simulink model "ap_12BAdapted_with_contracts_AutoPilot"  (R2017b)
settings: Solver=FixedStepDiscrete  StartTime=0.0  StopTime=500  FixedStep=Ts  RelTol=1e-3  EnableMultiTasking=on
undefined symbols (not defined in the file): beaver_b, beaver_c, beaver_mass, beaver_S, Cl0, Cl_alpha2_dpt, Cl_beta, Cl_da, Cl_da_alpha, Cl_dr, Cl_p, Cl_r, Cm0, Cm_alpha, Cm_alpha2, Cm_beta2, Cm_de, Cm_df, Cm_dpt, Cm_q, Cm_r, Cn0, Cn_beta, Cn_beta3, Cn_da, Cn_dpt3, Cn_dr, Cn_p, Cn_q, Cn_r, contractAfterSimulation, contractBeforeSimulation, ContractBlock, ContractEnsureBlock, ContractGuaranteeBlock, ContractModeBlock, ContractRequireBlock, ContractValidatorBlock, Cx0, Cx_alpha, Cx_alpha2, Cx_alpha3, Cx_df, Cx_df_alpha, Cx_dpt, Cx_dpt2_alpha, Cx_dr, Cx_q, Cy0, Cy_beta, Cy_da, Cy_dr, Cy_dr_alpha, Cy_p, Cy_r, Cz0, Cz_alpha, Cz_alpha3, Cz_de, Cz_de_beta ... (+32)
libraries: simulink x10, cocosimLibs x3
(part 3 of 4)

== system ap_12BAdapted_with_contracts_AutoPilot/GlobalScope/DeHavilland Beaver Airframe/Aircraft Dynamics/6DoF (Quaternion)/Calculate DCM & Euler Angles/Quaternions to Direction Cosine Matrix ==
  Quat : Inport  Unit=1  PortDimensions=4
  A11 : Subsystem
  A12 : Subsystem
  A13 : Subsystem
  A21 : Subsystem
  A22 : Subsystem
  A23 : Subsystem
  A31 : Subsystem
  A32 : Subsystem
  A33 : Subsystem
  Create 3x3 Matrix : Subsystem  mask(Create 3x3 Matrix){}
      mask help: shared_aeroblks:sharedaeroblkutil:blockCreate3x3MatrixDesc
      mask init:
      | if license('test','aerospace_blockset')
      |     aerosharedicon('shared');
      | elseif license('test','powertrain_blockset')
      |     sharedautoicon('shared');
      | end
      mask Help: eval('if license(''test'',''aerospace_blockset'')aerosharedhelp(''create_threebythree_matrix'');elseif license(''test'',''powertrain_blockset'')sharedautohelp(''create_threebythree_matrix'');end')
      mask Display:
      | port_label('input',1,'A_{11}','texmode','on');
      | port_label('input',2,'A_{12}','texmode','on');
      | port_label('input',3,'A_{13}','texmode','on');
      | port_label('input',4,'A_{21}','texmode','on');
      | port_label('input',5,'A_{22}','texmode','on');
      | port_label('input',6,'A_{23}','texmode','on');
      | port_label('input',7,'A_{31}','texmode','on');
      | port_label('input',8,'A_{32}','texmode','on');
      | port_label('input',9,'A_{33}','texmode','on');
      | port_label('output',1,'A','texmode','on');
  Quaternion Normalize : Subsystem  mask(Quaternion Normalize){}
      mask help: shared_aeroblks:sharedaeroblkutil:blockQuaternionNormalizeDesc
      mask init:
      | if license('test','aerospace_blockset')
      |     aerosharedicon('shared');
      | elseif license('test','powertrain_blockset')
      |     sharedautoicon('shared');
      | end
      mask Help: eval('if license(''test'',''aerospace_blockset'')aerosharedhelp;elseif license(''test'',''powertrain_blockset'')sharedautohelp;end')
  DCM : Outport  Unit=1  PortDimensions=[3,3]  VectorParamsAs1DForOutWhenUnconnected=off
  wires:
  A21/1(A21) -> Create 3x3 Matrix/4(M21)
  A12/1(A12) -> Create 3x3 Matrix/2(M12)
  Create 3x3 Matrix/1(Matrix) -> DCM/1
  A22/1(A22) -> Create 3x3 Matrix/5(M22)
  A32/1(A32) -> Create 3x3 Matrix/8(M32)
  A33/1(A33) -> Create 3x3 Matrix/9(M33)
  A31/1(A31) -> Create 3x3 Matrix/7(M31)
  A11/1(A11) -> Create 3x3 Matrix/1(M11)
  A13/1(A13) -> Create 3x3 Matrix/3(M13)
  A23/1(A23) -> Create 3x3 Matrix/6(M23)
  Quaternion Normalize/1(normal(q)) -> A11/1(normal(q)), A12/1(normal(q)), A13/1(normal(q)), A21/1(normal(q)), A22/1(normal(q)), A23/1(normal(q)), A31/1(normal(q)), A32/1(normal(q)), A33/1(normal(q))
  Quat/1 -> Quaternion Normalize/1(q)

== system ap_12BAdapted_with_contracts_AutoPilot/GlobalScope/DeHavilland Beaver Airframe/Aircraft Dynamics/6DoF (Quaternion)/Calculate DCM & Euler Angles/Quaternions to Rotation Angles (ZYX) ==
  q : Inport
  Quaternion Normalize : Subsystem
  Trigonometric Function1 : Trigonometry  Operator=atan2
  Trigonometric Function3 : Trigonometry  Operator=atan2
  Vector Concatenate : Concatenate  NumInputs=3
  fcn1 : Fcn  Expr=2*(u[2]*u[3] + u[1]*u[4])
  fcn2 : Fcn  Expr=u[1]*u[1] + u[2]*u[2] - u[3]*u[3] - u[4]*u[4]
  fcn3 : Fcn  Expr=-2*(u[2]*u[4] - u[1]*u[3])
  fcn4 : Fcn  Expr=2*(u[3]*u[4] + u[1]*u[2])
  fcn5 : Fcn  Expr=u[1]*u[1] - u[2]*u[2] - u[3]*u[3] + u[4]*u[4]
  trigFcn : Trigonometry  Operator=asin
  R1,R2,R3 : Outport  VectorParamsAs1DForOutWhenUnconnected=off
  wires:
  fcn5/1 -> Trigonometric Function3/2
  fcn4/1 -> Trigonometric Function3/1
  fcn2/1 -> Trigonometric Function1/2
  fcn3/1 -> trigFcn/1
  q/1 -> Quaternion Normalize/1(q)
  Vector Concatenate/1 -> R1,R2,R3/1
  Trigonometric Function3/1 -> Vector Concatenate/3  "r3"
  Trigonometric Function1/1 -> Vector Concatenate/1  "r1"
  Quaternion Normalize/1(normal(q)) -> fcn1/1, fcn2/1, fcn5/1, fcn4/1, fcn3/1
  trigFcn/1 -> Vector Concatenate/2  "r2"
  fcn1/1 -> Trigonometric Function1/1

== system ap_12BAdapted_with_contracts_AutoPilot/GlobalScope/DeHavilland Beaver Airframe/Aircraft Dynamics/6DoF (Quaternion)/Calculate DCM & Euler Angles/ResetIntegratorInternal1 ==
  note: ic
  note: Level Reset Integration With Saturation
      | y(n) = y(n-1) + K*Ts*u(n-1)
  U : Inport
  R : Inport  Port=2
  IC : Inport  Port=3
  Constant : Constant  Value=1.0
  Constant1 : Constant  Value=Ts
  Product : Product  RndMeth=Zero
  Product1 : Product  RndMeth=Zero
  Saturation : Saturate  UpperLimit=20  LowerLimit=-20
  Sum3 : Sum
  Switch : Switch  Criteria=u2 ~= 0
  Switch1 : Switch  Criteria=u2 ~= 0
  X : UnitDelay  SampleTime=Ts  HasFrameUpgradeWarning=on
  Y : Outport  VectorParamsAs1DForOutWhenUnconnected=off
  wires:
  Product1/1 -> Sum3/1
  U/1 -> Product1/2
  Sum3/1 -> Switch1/3
  Product/1 -> Product1/1
  Switch/1 -> Saturation/1
  IC/1 -> Switch1/1, Switch/1
  Constant1/1 -> Product/2  "deltaT"
  Switch1/1 -> X/1
  Constant/1 -> Product/1  "gain"
  Saturation/1 -> Y/1, Sum3/2
  R/1 -> Switch1/2, Switch/2
  X/1 -> Switch/3

== system ap_12BAdapted_with_contracts_AutoPilot/GlobalScope/DeHavilland Beaver Airframe/Aircraft Dynamics/6DoF (Quaternion)/Calculate DCM & Euler Angles/Rotation Angles to Quats (ZYX) ==
  "R1, R2, R3" : Inport
  1/2 : Gain  Gain=0.5  SaturateOnIntegerOverflow=on  OutDataTypeStr=Inherit: Same as input  ParamDataTypeStr=Inherit: Same as input
  Mux1 : Mux  Inputs=2
  Mux2 : Mux
  q0 : Fcn  Expr=u(4)*u(5)*u(6) + u(1)*u(2)*u(3)
  q1 : Fcn  Expr=u(4)*u(5)*u(3) - u(1)*u(2)*u(6)
  q2 : Fcn  Expr=u(4)*u(2)*u(6) + u(1)*u(5)*u(3)
  q3 : Fcn  Expr=u(1)*u(5)*u(6) - u(4)*u(2)*u(3)
  sincos : Trigonometry  Operator=sincos
  Quat : Outport  VectorParamsAs1DForOutWhenUnconnected=off
  wires:
  sincos/1 -> Mux1/1
  1/2/1 -> sincos/1
  "R1, R2, R3"/1 -> 1/2/1
  sincos/2 -> Mux1/2
  Mux1/1 -> q0/1, q1/1, q2/1, q3/1
  q1/1 -> Mux2/2
  q2/1 -> Mux2/3
  q3/1 -> Mux2/4
  Mux2/1 -> Quat/1
  q0/1 -> Mux2/1

== system ap_12BAdapted_with_contracts_AutoPilot/GlobalScope/DeHavilland Beaver Airframe/Aircraft Dynamics/6DoF (Quaternion)/Calculate DCM & Euler Angles/ic3 ==
  ic : Inport
  Constant : Constant  Value=0
  Unit Delay : UnitDelay  InitialCondition=1  SampleTime=-1  HasFrameUpgradeWarning=on
  R : Outport  VectorParamsAs1DForOutWhenUnconnected=off
  IC : Outport  Port=2  VectorParamsAs1DForOutWhenUnconnected=off
  wires:
  Constant/1 -> Unit Delay/1
  Unit Delay/1 -> R/1
  ic/1 -> IC/1

== system ap_12BAdapted_with_contracts_AutoPilot/GlobalScope/DeHavilland Beaver Airframe/Aircraft Dynamics/6DoF (Quaternion)/Calculate DCM & Euler Angles/qd ==
  p q r : Inport
  q0 q1 q2 q3 : Inport  Port=2
  Constant : Constant
  Dot Product : DotProduct  OutDataTypeStr=Inherit: Inherit via internal rule
  High Gain Quaternion Normalization : Gain  Gain=1.0  SaturateOnIntegerOverflow=on  OutDataTypeStr=Inherit: Same as input  ParamDataTypeStr=Inherit: Same as input
  Mux1 : Mux  Inputs=[3 4 1]
  Mux2 : Mux
  Sum : Sum  Inputs=|+-  SaturateOnIntegerOverflow=on  InputSameDT=on  OutDataTypeStr=Inherit: Same as first input
  q0dot : Fcn  Expr=-0.5 * ( u[5]*u[1]+u[6]*u[2]+u[7]*u[3] ) + u[8]*u[4]
  q1dot : Fcn  Expr=0.5 * ( u[4]*u[1]+u[6]*u[3]-u[7]*u[2] ) + u[8]*u[5]
  q2dot : Fcn  Expr=0.5 * ( u[4]*u[2]+u[7]*u[1]-u[5]*u[3] ) + u[8]*u[6]
  q3dot : Fcn  Expr=0.5 * ( u[4]*u[3]+u[5]*u[2]-u[6]*u[1] ) + u[8]*u[7]
  qdot : Outport  VectorParamsAs1DForOutWhenUnconnected=off
  wires:
  p q r/1 -> Mux1/1
  q3dot/1 -> Mux2/4
  q2dot/1 -> Mux2/3
  q1dot/1 -> Mux2/2
  Constant/1 -> Sum/1
  Mux1/1 -> q2dot/1, q3dot/1, q0dot/1, q1dot/1
  q0dot/1 -> Mux2/1
  Mux2/1 -> qdot/1
  Sum/1 -> High Gain Quaternion Normalization/1
  Dot Product/1 -> Sum/2
  High Gain Quaternion Normalization/1 -> Mux1/3
  q0 q1 q2 q3/1 -> Dot Product/1, Dot Product/2, Mux1/2

== system ap_12BAdapted_with_contracts_AutoPilot/GlobalScope/DeHavilland Beaver Airframe/Aircraft Dynamics/6DoF (Quaternion)/Calculate omega_dot/3x3 CrossProduct ==
  A : Inport
  B : Inport  Port=2
  "A " : InportShadow
  "B " : InportShadow  Port=2
  Subsystem : Subsystem
  Subsystem1 : Subsystem
  Sum : Sum  Inputs=+|-  SaturateOnIntegerOverflow=on  InputSameDT=on  OutDataTypeStr=Inherit: Same as first input
  C : Outport  VectorParamsAs1DForOutWhenUnconnected=off
  wires:
  "A "/1 -> Subsystem1/1(A)
  Subsystem/1(Out1) -> Sum/1
  B/1 -> Subsystem/2(B)
  Sum/1 -> C/1
  "B "/1 -> Subsystem1/2(B)
  Subsystem1/1(Out1) -> Sum/2
  A/1 -> Subsystem/1(A)

== system ap_12BAdapted_with_contracts_AutoPilot/GlobalScope/DeHavilland Beaver Airframe/Aircraft Dynamics/6DoF (Quaternion)/Calculate omega_dot/I x w ==
  p q r : Inport
  Inertia : Inport  Port=2
  Product : Product  Multiplication=Matrix(*)  SaturateOnIntegerOverflow=on  InputSameDT=on  OutDataTypeStr=Inherit: Same as first input
  Reshape1 : Reshape  OutputDimensionality=Column vector (2-D)
  Reshape2 : Reshape
  I * w : Outport  VectorParamsAs1DForOutWhenUnconnected=off
  wires:
  Reshape2/1 -> I * w/1
  Reshape1/1 -> Product/2
  p q r/1 -> Reshape1/1
  Inertia/1 -> Product/1
  Product/1 -> Reshape2/1

== system ap_12BAdapted_with_contracts_AutoPilot/GlobalScope/DeHavilland Beaver Airframe/Aircraft Dynamics/6DoF (Quaternion)/Calculate omega_dot/I x w1 ==
  I_dot : Inport
  p q r : Inport  Port=2
  Product : Product  Multiplication=Matrix(*)  SaturateOnIntegerOverflow=on  InputSameDT=on  OutDataTypeStr=Inherit: Same as first input
  Reshape1 : Reshape  OutputDimensionality=Column vector (2-D)
  Reshape2 : Reshape
  Id * w : Outport  VectorParamsAs1DForOutWhenUnconnected=off
  wires:
  Reshape2/1 -> Id * w/1
  Reshape1/1 -> Product/2
  Product/1 -> Reshape2/1
  I_dot/1 -> Product/1
  p q r/1 -> Reshape1/1

== system ap_12BAdapted_with_contracts_AutoPilot/GlobalScope/DeHavilland Beaver Airframe/Aircraft Dynamics/Total Forces and Moments/Actuators/sof ==
  Ac_dem : Inport
  2*zeta * wn : Gain  Gain=2.0 * z_fin* wn_fin  SaturateOnIntegerOverflow=on  OutDataTypeStr=Inherit: Same as input  ParamDataTypeStr=Inherit: Same as input
  Demand limits : Saturate  UpperLimit=fin_max  LowerLimit=fin_min
  ResetIntegratorInternal : Subsystem
  ResetIntegratorInternal1 : Subsystem
  Sum2 : Sum  Inputs=|+-  SaturateOnIntegerOverflow=on  InputSameDT=on  OutDataTypeStr=Inherit: Same as first input
  Sum3 : Sum  Inputs=|+-  SaturateOnIntegerOverflow=on  InputSameDT=on  OutDataTypeStr=Inherit: Same as first input
  ic1 : Subsystem
  ic3 : Subsystem
  rate limit*2*zeta/wn : Saturate  UpperLimit=fin_maxrate*2*z_fin/wn_fin  LowerLimit=-fin_maxrate*2*z_fin/wn_fin
  wn^2 : Gain  Gain=wn_fin* wn_fin  SaturateOnIntegerOverflow=on  OutDataTypeStr=Inherit: Same as input  ParamDataTypeStr=Inherit: Same as input
  Ac_ac : Outport  VectorParamsAs1DForOutWhenUnconnected=off
  wires:
  ResetIntegratorInternal1/1(Y) -> Ac_ac/1, Sum3/2
  wn^2/1 -> Sum2/1
  ResetIntegratorInternal/1(Y) -> ResetIntegratorInternal1/1(U), 2*zeta * wn/1
  Sum2/1 -> ResetIntegratorInternal/1(U)
  Demand limits/1 -> Sum3/1
  rate limit*2*zeta/wn/1 -> wn^2/1
  Ac_dem/1 -> Demand limits/1
  Sum3/1 -> rate limit*2*zeta/wn/1
  2*zeta * wn/1 -> Sum2/2
  ic3/2(IC) -> ResetIntegratorInternal/3(ic)
  ic3/1(R) -> ResetIntegratorInternal/2(R)
  ic1/1(R) -> ResetIntegratorInternal1/2(R)
  ic1/2(IC) -> ResetIntegratorInternal1/3(ic)

== system ap_12BAdapted_with_contracts_AutoPilot/GlobalScope/DeHavilland Beaver Airframe/Aircraft Dynamics/Total Forces and Moments/Actuators/sof1 ==
  Ac_dem : Inport
  2*zeta * wn : Gain  Gain=2.0 * z_fin* wn_fin  SaturateOnIntegerOverflow=on  OutDataTypeStr=Inherit: Same as input  ParamDataTypeStr=Inherit: Same as input
  Demand limits : Saturate  UpperLimit=fin_max  LowerLimit=fin_min
  ResetIntegratorInternal : Subsystem
  ResetIntegratorInternal1 : Subsystem
  Sum2 : Sum  Inputs=|+-  SaturateOnIntegerOverflow=on  InputSameDT=on  OutDataTypeStr=Inherit: Same as first input
  Sum3 : Sum  Inputs=|+-  SaturateOnIntegerOverflow=on  InputSameDT=on  OutDataTypeStr=Inherit: Same as first input
  ic1 : Subsystem
  ic3 : Subsystem
  rate limit*2*zeta/wn : Saturate  UpperLimit=fin_maxrate*2*z_fin/wn_fin  LowerLimit=-fin_maxrate*2*z_fin/wn_fin
  wn^2 : Gain  Gain=wn_fin* wn_fin  SaturateOnIntegerOverflow=on  OutDataTypeStr=Inherit: Same as input  ParamDataTypeStr=Inherit: Same as input
  Ac_ac : Outport  VectorParamsAs1DForOutWhenUnconnected=off
  wires:
  ic1/2(IC) -> ResetIntegratorInternal1/3(ic)
  ic1/1(R) -> ResetIntegratorInternal1/2(R)
  ic3/1(R) -> ResetIntegratorInternal/2(R)
  ic3/2(IC) -> ResetIntegratorInternal/3(ic)
  2*zeta * wn/1 -> Sum2/2
  Sum3/1 -> rate limit*2*zeta/wn/1
  Ac_dem/1 -> Demand limits/1
  rate limit*2*zeta/wn/1 -> wn^2/1
  Demand limits/1 -> Sum3/1
  Sum2/1 -> ResetIntegratorInternal/1(U)
  ResetIntegratorInternal/1(Y) -> 2*zeta * wn/1, ResetIntegratorInternal1/1(U)
  wn^2/1 -> Sum2/1
  ResetIntegratorInternal1/1(Y) -> Sum3/2, Ac_ac/1

== system ap_12BAdapted_with_contracts_AutoPilot/GlobalScope/DeHavilland Beaver Airframe/Aircraft Dynamics/Total Forces and Moments/Actuators/sof2 ==
  Ac_dem : Inport
  2*zeta * wn : Gain  Gain=2.0 * z_fin* wn_fin  SaturateOnIntegerOverflow=on  OutDataTypeStr=Inherit: Same as input  ParamDataTypeStr=Inherit: Same as input
  Demand limits : Saturate  UpperLimit=fin_max  LowerLimit=fin_min
  ResetIntegratorInternal : Subsystem
  ResetIntegratorInternal1 : Subsystem
  Sum2 : Sum  Inputs=|+-  SaturateOnIntegerOverflow=on  InputSameDT=on  OutDataTypeStr=Inherit: Same as first input
  Sum3 : Sum  Inputs=|+-  SaturateOnIntegerOverflow=on  InputSameDT=on  OutDataTypeStr=Inherit: Same as first input
  ic1 : Subsystem
  ic3 : Subsystem
  rate limit*2*zeta/wn : Saturate  UpperLimit=fin_maxrate*2*z_fin/wn_fin  LowerLimit=-fin_maxrate*2*z_fin/wn_fin
  wn^2 : Gain  Gain=wn_fin* wn_fin  SaturateOnIntegerOverflow=on  OutDataTypeStr=Inherit: Same as input  ParamDataTypeStr=Inherit: Same as input
  Ac_ac : Outport  VectorParamsAs1DForOutWhenUnconnected=off
  wires:
  ResetIntegratorInternal1/1(Y) -> Ac_ac/1, Sum3/2
  wn^2/1 -> Sum2/1
  ResetIntegratorInternal/1(Y) -> ResetIntegratorInternal1/1(U), 2*zeta * wn/1
  Sum2/1 -> ResetIntegratorInternal/1(U)
  Demand limits/1 -> Sum3/1
  rate limit*2*zeta/wn/1 -> wn^2/1
  Ac_dem/1 -> Demand limits/1
  Sum3/1 -> rate limit*2*zeta/wn/1
  2*zeta * wn/1 -> Sum2/2
  ic3/2(IC) -> ResetIntegratorInternal/3(ic)
  ic3/1(R) -> ResetIntegratorInternal/2(R)
  ic1/1(R) -> ResetIntegratorInternal1/2(R)
  ic1/2(IC) -> ResetIntegratorInternal1/3(ic)

== system ap_12BAdapted_with_contracts_AutoPilot/GlobalScope/DeHavilland Beaver Airframe/Aircraft Dynamics/Total Forces and Moments/Aerodynamics/Actuator Increments ==
  alpha : Inport
  beta : Inport  Port=2
  Actuator Deflections : Inport  Port=3
  Aileron : Subsystem
  Elevator : Subsystem
  Flap : Subsystem
  Rudder : Subsystem
  Sum1 : Sum  SaturateOnIntegerOverflow=on
  Sum2 : Sum  SaturateOnIntegerOverflow=on
  Sum3 : Sum  SaturateOnIntegerOverflow=on
  Coefficients : Outport  VectorParamsAs1DForOutWhenUnconnected=off
  wires:
  Actuator Deflections/1 -> Flap/2(Actuators), Aileron/2(Actuators), Elevator/1(Actuators), Rudder/2(Actuators)
  alpha/1 -> Flap/1(Alpha), Rudder/1(Alpha), Aileron/1(alpha)
  beta/1 -> Elevator/2(Beta)
  Aileron/1(delCoeff) -> Sum1/1
  Elevator/1(delCoeff) -> Sum1/2
  Rudder/1(delCoeff) -> Sum2/2
  Flap/1(delCoeff) -> Sum3/2
  Sum3/1 -> Coefficients/1
  Sum1/1 -> Sum2/1
  Sum2/1 -> Sum3/1

== system ap_12BAdapted_with_contracts_AutoPilot/GlobalScope/DeHavilland Beaver Airframe/Aircraft Dynamics/Total Forces and Moments/Aerodynamics/Body Rate Damping ==
  V : Inport
  p,q,r : Inport  Port=2
  Demux : Demux  Outputs=3
  Product : Product  SaturateOnIntegerOverflow=on  InputSameDT=on  OutDataTypeStr=Inherit: Same as first input
  Product1 : Product  SaturateOnIntegerOverflow=on  InputSameDT=on  OutDataTypeStr=Inherit: Same as first input
  Product2 : Product  SaturateOnIntegerOverflow=on  InputSameDT=on  OutDataTypeStr=Inherit: Same as first input
  Product3 : Product  Inputs=*/  SaturateOnIntegerOverflow=on  InputSameDT=on  OutDataTypeStr=Inherit: Same as first input
  Reference Length : Gain  Gain=beaver_c  SaturateOnIntegerOverflow=on  OutDataTypeStr=Inherit: Same as input  ParamDataTypeStr=Inherit: Same as input
  Reference Span : Gain  Gain=beaver_b/2  SaturateOnIntegerOverflow=on  OutDataTypeStr=Inherit: Same as input  ParamDataTypeStr=Inherit: Same as input
  "Reference Span " : Gain  Gain=beaver_b/2  SaturateOnIntegerOverflow=on  OutDataTypeStr=Inherit: Same as input  ParamDataTypeStr=Inherit: Same as input
  Sum1 : Sum  SaturateOnIntegerOverflow=on
  Sum2 : Sum  SaturateOnIntegerOverflow=on
  p : Subsystem
  q : Subsystem
  r : Subsystem
  Coefficients : Outport  VectorParamsAs1DForOutWhenUnconnected=off
  wires:
  p/1(delCoeff) -> Product/1
  q/1(delCoeff) -> Product1/1
  p,q,r/1 -> Demux/1
  Demux/1 -> Product/2  "p"
  Demux/2 -> Product1/2  "q"
  Demux/3 -> Product2/2  "r"
  Sum1/1 -> Product3/1
  V/1 -> Product3/2
  Product3/1 -> Coefficients/1
  Product1/1 -> Reference Length/1
  Product2/1 -> "Reference Span "/1
  Product/1 -> Reference Span/1
  r/1(delCoeff) -> Product2/1
  Reference Length/1 -> Sum2/2
  "Reference Span "/1 -> Sum1/2
  Reference Span/1 -> Sum2/1
  Sum2/1 -> Sum1/1

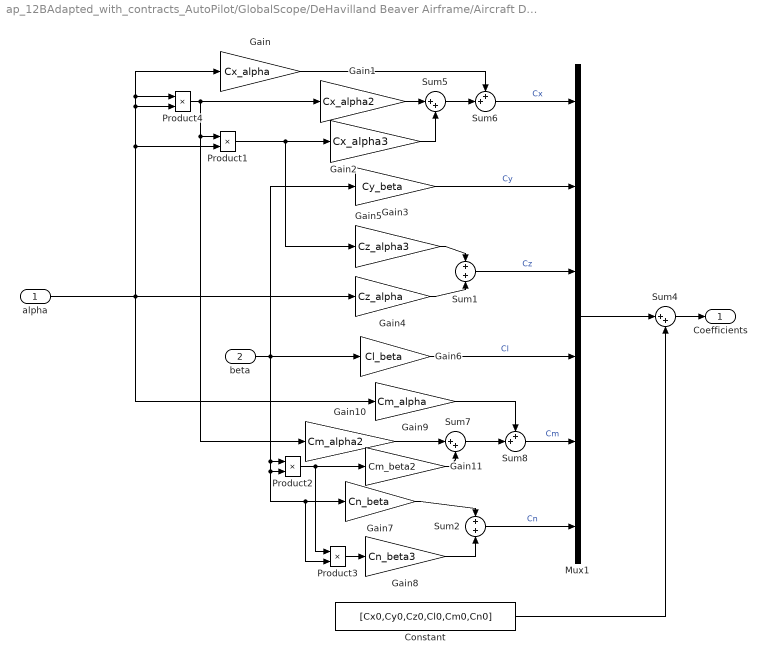
== system ap_12BAdapted_with_contracts_AutoPilot/GlobalScope/DeHavilland Beaver Airframe/Aircraft Dynamics/Total Forces and Moments/Aerodynamics/Datum Coefficients ==
  alpha : Inport
  beta : Inport  Port=2
  Constant : Constant  Value=[Cx0,Cy0,Cz0,Cl0,Cm0,Cn0]
  Gain : Gain  Gain=Cx_alpha  SaturateOnIntegerOverflow=on  OutDataTypeStr=Inherit: Same as input  ParamDataTypeStr=Inherit: Same as input
  Gain1 : Gain  Gain=Cx_alpha2  SaturateOnIntegerOverflow=on  OutDataTypeStr=Inherit: Same as input  ParamDataTypeStr=Inherit: Same as input
  Gain10 : Gain  Gain=Cm_alpha2  SaturateOnIntegerOverflow=on  OutDataTypeStr=Inherit: Same as input  ParamDataTypeStr=Inherit: Same as input
  Gain11 : Gain  Gain=Cm_beta2  SaturateOnIntegerOverflow=on  OutDataTypeStr=Inherit: Same as input  ParamDataTypeStr=Inherit: Same as input
  Gain2 : Gain  Gain=Cx_alpha3  SaturateOnIntegerOverflow=on  OutDataTypeStr=Inherit: Same as input  ParamDataTypeStr=Inherit: Same as input
  Gain3 : Gain  Gain=Cy_beta  SaturateOnIntegerOverflow=on  OutDataTypeStr=Inherit: Same as input  ParamDataTypeStr=Inherit: Same as input
  Gain4 : Gain  Gain=Cz_alpha  SaturateOnIntegerOverflow=on  OutDataTypeStr=Inherit: Same as input  ParamDataTypeStr=Inherit: Same as input
  Gain5 : Gain  Gain=Cz_alpha3  SaturateOnIntegerOverflow=on  OutDataTypeStr=Inherit: Same as input  ParamDataTypeStr=Inherit: Same as input
  Gain6 : Gain  Gain=Cl_beta  SaturateOnIntegerOverflow=on  OutDataTypeStr=Inherit: Same as input  ParamDataTypeStr=Inherit: Same as input
  Gain7 : Gain  Gain=Cn_beta  SaturateOnIntegerOverflow=on  OutDataTypeStr=Inherit: Same as input  ParamDataTypeStr=Inherit: Same as input
  Gain8 : Gain  Gain=Cn_beta3  SaturateOnIntegerOverflow=on  OutDataTypeStr=Inherit: Same as input  ParamDataTypeStr=Inherit: Same as input
  Gain9 : Gain  Gain=Cm_alpha  SaturateOnIntegerOverflow=on  OutDataTypeStr=Inherit: Same as input  ParamDataTypeStr=Inherit: Same as input
  Mux1 : Mux  Inputs=6
  Product{1..4} (4 alike) : Product  SaturateOnIntegerOverflow=on  InputSameDT=on  OutDataTypeStr=Inherit: Same as first input
  Sum1 : Sum  SaturateOnIntegerOverflow=on
  Sum2 : Sum  SaturateOnIntegerOverflow=on
  Sum4 : Sum  Inputs=|++  SaturateOnIntegerOverflow=on
  Sum5 : Sum  Inputs=|++  SaturateOnIntegerOverflow=on
  Sum6 : Sum  Inputs=++|  SaturateOnIntegerOverflow=on
  Sum7 : Sum  Inputs=|++  SaturateOnIntegerOverflow=on
  Sum8 : Sum  Inputs=++|  SaturateOnIntegerOverflow=on
  Coefficients : Outport  VectorParamsAs1DForOutWhenUnconnected=off
  wires:
  Constant/1 -> Sum4/2
  Sum4/1 -> Coefficients/1
  Mux1/1 -> Sum4/1
  Gain10/1 -> Sum7/1
  Product2/1 -> Product3/1, Gain11/1
  Gain11/1 -> Sum7/2
  Gain9/1 -> Sum8/1
  Sum8/1 -> Mux1/5  "Cm"
  Product3/1 -> Gain8/1
  Gain8/1 -> Sum2/2
  Gain7/1 -> Sum2/1
  Gain5/1 -> Sum1/1
  Gain4/1 -> Sum1/2
  Product1/1 -> Gain5/1, Gain2/1
  Product4/1 -> Product1/1, Gain10/1, Gain1/1
  Gain/1 -> Sum6/1
  Sum2/1 -> Mux1/6  "Cn"
  Sum6/1 -> Mux1/1  "Cx"
  Sum1/1 -> Mux1/3  "Cz"
  Gain3/1 -> Mux1/2  "Cy"
  Gain6/1 -> Mux1/4  "Cl"
  alpha/1 -> Product1/2, Product4/2, Product4/1, Gain/1, Gain9/1, Gain4/1
  beta/1 -> Gain6/1, Gain3/1, Product3/2, Gain7/1, Product2/2, Product2/1
  Gain1/1 -> Sum5/1
  Gain2/1 -> Sum5/2
  Sum5/1 -> Sum6/2
  Sum7/1 -> Sum8/2

== system ap_12BAdapted_with_contracts_AutoPilot/GlobalScope/DeHavilland Beaver Airframe/Aircraft Dynamics/Total Forces and Moments/Engine /eng ==
  note: dpt
  dpt : Inport
  alpha : Inport  Port=2
  Constant : Constant  Value=0
  Gain1 : Gain  Gain=Cn_dpt3  SaturateOnIntegerOverflow=on  OutDataTypeStr=Inherit: Same as input  ParamDataTypeStr=Inherit: Same as input
  Gain2 : Gain  Gain=Cm_dpt  SaturateOnIntegerOverflow=on  OutDataTypeStr=Inherit: Same as input  ParamDataTypeStr=Inherit: Same as input
  Gain3 : Gain  Gain=Cl_alpha2_dpt  SaturateOnIntegerOverflow=on  OutDataTypeStr=Inherit: Same as input  ParamDataTypeStr=Inherit: Same as input
  Gain4 : Gain  Gain=Cz_dpt  SaturateOnIntegerOverflow=on  OutDataTypeStr=Inherit: Same as input  ParamDataTypeStr=Inherit: Same as input
  Gain5 : Gain  Gain=Cx_dpt  SaturateOnIntegerOverflow=on  OutDataTypeStr=Inherit: Same as input  ParamDataTypeStr=Inherit: Same as input
  Gain6 : Gain  Gain=Cx_dpt2_alpha  SaturateOnIntegerOverflow=on  OutDataTypeStr=Inherit: Same as input  ParamDataTypeStr=Inherit: Same as input
  Mux2 : Mux  Inputs=6
  Product{,1..4,6} (6 alike) : Product  SaturateOnIntegerOverflow=on  OutDataTypeStr=Inherit: Same as first input
  Sum : Sum  Inputs=|++  SaturateOnIntegerOverflow=on
  Cprop : Outport  VectorParamsAs1DForOutWhenUnconnected=off
  wires:
  Sum/1 -> Mux2/1
  Gain6/1 -> Sum/2
  Gain5/1 -> Sum/1
  Constant/1 -> Mux2/2
  Gain4/1 -> Mux2/3
  Gain3/1 -> Mux2/4
  Gain2/1 -> Mux2/5
  Gain1/1 -> Mux2/6
  Product4/1 -> Gain3/1
  Product2/1 -> Gain6/1
  dpt/1 -> Gain5/1, Product/1, Product/2, Product6/2, Product1/2, Product1/1, Gain2/1, Gain4/1, Product4/2
  alpha/1 -> Product2/2, Product3/1, Product3/2
  Mux2/1 -> Cprop/1  "Cprop"
  Product/1 -> Product2/1
  Product3/1 -> Product4/1
  Product1/1 -> Product6/1
  Product6/1 -> Gain1/1

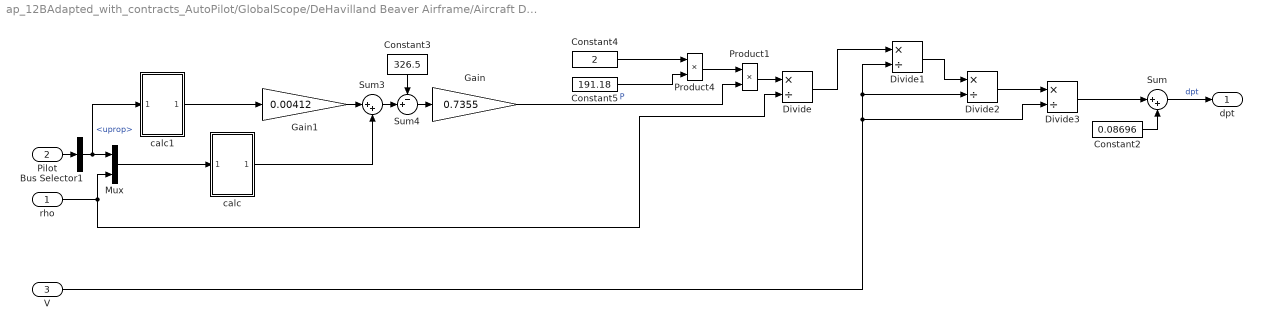
== system ap_12BAdapted_with_contracts_AutoPilot/GlobalScope/DeHavilland Beaver Airframe/Aircraft Dynamics/Total Forces and Moments/Engine /pow ==
  rho : Inport
  Pilot : Inport  Port=2
  V : Inport  Port=3
  Bus Selector1 : BusSelector  OutputSignals=uprop
  Constant2 : Constant  Value=0.08696
  Constant3 : Constant  Value=326.5
  Constant4 : Constant  Value=2
  Constant5 : Constant  Value=191.18
  Divide{,1..3} (4 alike) : Product  Inputs=*/
  Gain : Gain  Gain=0.7355  SaturateOnIntegerOverflow=on  OutDataTypeStr=Inherit: Same as input  ParamDataTypeStr=Inherit: Same as input
  Gain1 : Gain  Gain=0.00412  SaturateOnIntegerOverflow=on  OutDataTypeStr=Inherit: Same as input  ParamDataTypeStr=Inherit: Same as input
  Mux : Mux  Inputs=2
  Product1 : Product  SaturateOnIntegerOverflow=on  OutDataTypeStr=Inherit: Same as first input
  Product4 : Product  SaturateOnIntegerOverflow=on  OutDataTypeStr=Inherit: Same as first input
  Sum : Sum  Inputs=|++  SaturateOnIntegerOverflow=on
  Sum3 : Sum  Inputs=|++  SaturateOnIntegerOverflow=on
  Sum4 : Sum  Inputs=-+|  SaturateOnIntegerOverflow=on
  calc : Subsystem
  calc1 : Subsystem
  dpt : Outport  VectorParamsAs1DForOutWhenUnconnected=off
  wires:
  calc/1(Out1) -> Sum3/2
  Constant3/1 -> Sum4/1
  Gain1/1 -> Sum3/1
  rho/1 -> Divide/2, Mux/2
  Sum/1 -> dpt/1  "dpt"
  V/1 -> Divide3/2, Divide1/2, Divide2/2
  Bus Selector1/1 -> calc1/1(In1), Mux/1  "<uprop>"
  Divide3/1 -> Sum/1
  Constant2/1 -> Sum/2
  Pilot/1 -> Bus Selector1/1
  Sum4/1 -> Gain/1
  Sum3/1 -> Sum4/2
  Mux/1 -> calc/1(In1)
  calc1/1(Out1) -> Gain1/1
  Constant4/1 -> Product4/1
  Constant5/1 -> Product4/2
  Product4/1 -> Product1/1
  Gain/1 -> Product1/2  "P"
  Product1/1 -> Divide/1
  Divide/1 -> Divide1/1
  Divide1/1 -> Divide2/1
  Divide2/1 -> Divide3/1

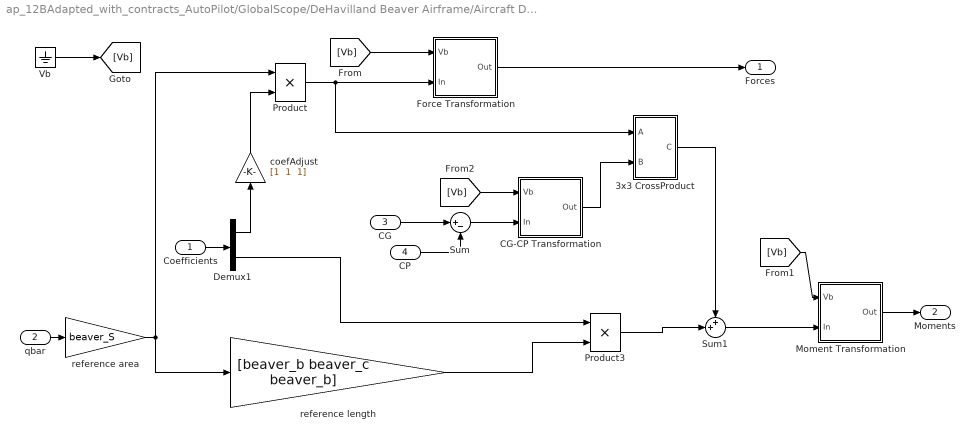
== system ap_12BAdapted_with_contracts_AutoPilot/GlobalScope/DeHavilland Beaver Airframe/Aircraft Dynamics/Total Forces and Moments/Forces and Moments/Aero F&M ==
  Coefficients : Inport
  qbar : Inport  Port=2
  CG : Inport  Port=3
  CP : Inport  Port=4
  3x3 CrossProduct : Subsystem
  CG-CP Transformation : Subsystem  mask(Passive){}
      mask init:
      | %aeroicon('aeroblk');
  Demux1 : Demux  Outputs=[3,3]
  Force Transformation : Subsystem  mask(Passive){}
      mask init:
      | %aeroicon('aeroblk');
  Moment Transformation : Subsystem  mask(Passive){}
      mask init:
      | %aeroicon('aeroblk');
  Product : Product  SaturateOnIntegerOverflow=on  InputSameDT=on  OutDataTypeStr=Inherit: Same as first input
  Product3 : Product  SaturateOnIntegerOverflow=on  InputSameDT=on  OutDataTypeStr=Inherit: Same as first input
  Sum : Sum  Inputs=|+-  SaturateOnIntegerOverflow=on
  Sum1 : Sum  Inputs=++|  SaturateOnIntegerOverflow=on  InputSameDT=on  OutDataTypeStr=Inherit: Same as first input
  Vb : Ground
  coefAdjust : Gain  Gain="[1  1  1]"
  reference area : Gain  Gain=beaver_S  SaturateOnIntegerOverflow=on  OutDataTypeStr=Inherit: Same as input  ParamDataTypeStr=Inherit: Same as input
  reference length : Gain  Gain=[beaver_b beaver_c beaver_b]  SaturateOnIntegerOverflow=on  OutDataTypeStr=Inherit: Same as input  ParamDataTypeStr=Inherit: Same as input
  Forces : Outport  VectorParamsAs1DForOutWhenUnconnected=off
  Moments : Outport  Port=2  VectorParamsAs1DForOutWhenUnconnected=off
  wires:
  [Vb] -> Force Transformation/1(Vb)
  CP/1 -> Sum/2
  reference length/1 -> Product3/2
  Demux1/2 -> Product3/1
  qbar/1 -> reference area/1
  coefAdjust/1 -> Product/2
  Force Transformation/1(Out) -> Forces/1
  Demux1/1 -> coefAdjust/1
  Coefficients/1 -> Demux1/1
  [Vb] -> Moment Transformation/1(Vb)
  [Vb] -> CG-CP Transformation/1(Vb)
  CG-CP Transformation/1(Out) -> 3x3 CrossProduct/2(B)
  Product3/1 -> Sum1/2
  Vb/1 -> [Vb]
  reference area/1 -> reference length/1, Product/1
  Moment Transformation/1(Out) -> Moments/1
  Product/1 -> 3x3 CrossProduct/1(A), Force Transformation/2(In)
  Sum/1 -> CG-CP Transformation/2(In)
  Sum1/1 -> Moment Transformation/2(In)
  3x3 CrossProduct/1(C) -> Sum1/1
  CG/1 -> Sum/1

== system ap_12BAdapted_with_contracts_AutoPilot/GlobalScope/DeHavilland Beaver Airframe/Aircraft Dynamics/6DoF (Quaternion)/Calculate DCM & Euler Angles/Quaternions to Direction Cosine Matrix/A11 ==
  normal(q) : Inport
  Demux : Demux
  Product{,1..3} (4 alike) : Product  RndMeth=Zero
  Sum : Sum  Inputs=++--
  A11 : Outport  VectorParamsAs1DForOutWhenUnconnected=off
  wires:
  Sum/1 -> A11/1
  Demux/4 -> Product/2, Product/1
  Demux/3 -> Product1/2, Product1/1
  Demux/2 -> Product2/2, Product2/1
  Demux/1 -> Product3/2, Product3/1
  Product3/1 -> Sum/1
  Product2/1 -> Sum/2
  Product1/1 -> Sum/3
  Product/1 -> Sum/4
  normal(q)/1 -> Demux/1

== system ap_12BAdapted_with_contracts_AutoPilot/GlobalScope/DeHavilland Beaver Airframe/Aircraft Dynamics/6DoF (Quaternion)/Calculate DCM & Euler Angles/Quaternions to Direction Cosine Matrix/A12 ==
  normal(q) : Inport
  Demux : Demux
  Gain : Gain  Gain=2
  Product2 : Product  RndMeth=Zero
  Product3 : Product  RndMeth=Zero
  Sum : Sum  Inputs=|++
  A12 : Outport  VectorParamsAs1DForOutWhenUnconnected=off
  wires:
  Product2/1 -> Sum/2
  Product3/1 -> Sum/1
  Sum/1 -> Gain/1
  Demux/1 -> Product3/2
  Demux/2 -> Product2/1
  Demux/4 -> Product3/1
  Demux/3 -> Product2/2
  normal(q)/1 -> Demux/1
  Gain/1 -> A12/1

== system ap_12BAdapted_with_contracts_AutoPilot/GlobalScope/DeHavilland Beaver Airframe/Aircraft Dynamics/6DoF (Quaternion)/Calculate DCM & Euler Angles/Quaternions to Direction Cosine Matrix/A13 ==
  normal(q) : Inport
  Demux : Demux
  Gain : Gain  Gain=2
  Product1 : Product  RndMeth=Zero
  Product2 : Product  RndMeth=Zero
  Sum : Sum  Inputs=|-+
  A13 : Outport  VectorParamsAs1DForOutWhenUnconnected=off
  wires:
  Demux/1 -> Product1/1
  Product1/1 -> Sum/1
  Product2/1 -> Sum/2
  Demux/4 -> Product2/2
  Demux/2 -> Product2/1
  Demux/3 -> Product1/2
  normal(q)/1 -> Demux/1
  Gain/1 -> A13/1
  Sum/1 -> Gain/1

== system ap_12BAdapted_with_contracts_AutoPilot/GlobalScope/DeHavilland Beaver Airframe/Aircraft Dynamics/6DoF (Quaternion)/Calculate DCM & Euler Angles/Quaternions to Direction Cosine Matrix/A21 ==
  normal(q) : Inport
  Demux : Demux
  Gain : Gain  Gain=2
  Product2 : Product  RndMeth=Zero
  Product3 : Product  RndMeth=Zero
  Sum : Sum  Inputs=|-+
  A21 : Outport  VectorParamsAs1DForOutWhenUnconnected=off
  wires:
  Gain/1 -> A21/1
  normal(q)/1 -> Demux/1
  Demux/3 -> Product2/2
  Demux/4 -> Product3/1
  Demux/2 -> Product2/1
  Demux/1 -> Product3/2
  Sum/1 -> Gain/1
  Product3/1 -> Sum/1
  Product2/1 -> Sum/2

== system ap_12BAdapted_with_contracts_AutoPilot/GlobalScope/DeHavilland Beaver Airframe/Aircraft Dynamics/6DoF (Quaternion)/Calculate DCM & Euler Angles/Quaternions to Direction Cosine Matrix/A22 ==
  normal(q) : Inport
  Demux : Demux
  Product{,1..3} (4 alike) : Product  RndMeth=Zero
  Sum : Sum  Inputs=+-+-
  A22 : Outport  VectorParamsAs1DForOutWhenUnconnected=off
  wires:
  normal(q)/1 -> Demux/1
  Product/1 -> Sum/4
  Product1/1 -> Sum/3
  Product2/1 -> Sum/2
  Product3/1 -> Sum/1
  Demux/1 -> Product3/1, Product3/2
  Demux/2 -> Product2/1, Product2/2
  Demux/3 -> Product1/1, Product1/2
  Demux/4 -> Product/1, Product/2
  Sum/1 -> A22/1

== system ap_12BAdapted_with_contracts_AutoPilot/GlobalScope/DeHavilland Beaver Airframe/Aircraft Dynamics/6DoF (Quaternion)/Calculate DCM & Euler Angles/Quaternions to Direction Cosine Matrix/A23 ==
  normal(q) : Inport
  Demux : Demux
  Gain : Gain  Gain=2
  Product1 : Product  RndMeth=Zero
  Product2 : Product  RndMeth=Zero
  Sum : Sum  Inputs=|++
  A23 : Outport  VectorParamsAs1DForOutWhenUnconnected=off
  wires:
  Demux/4 -> Product2/2
  Product2/1 -> Sum/2
  Product1/1 -> Sum/1
  Sum/1 -> Gain/1
  Demux/1 -> Product1/1
  Demux/2 -> Product1/2
  Demux/3 -> Product2/1
  Gain/1 -> A23/1
  normal(q)/1 -> Demux/1

== system ap_12BAdapted_with_contracts_AutoPilot/GlobalScope/DeHavilland Beaver Airframe/Aircraft Dynamics/6DoF (Quaternion)/Calculate DCM & Euler Angles/Quaternions to Direction Cosine Matrix/A31 ==
  normal(q) : Inport
  Demux : Demux
  Gain : Gain  Gain=2
  Product1 : Product  RndMeth=Zero
  Product2 : Product  RndMeth=Zero
  Sum : Sum  Inputs=|++
  A31 : Outport  VectorParamsAs1DForOutWhenUnconnected=off
  wires:
  Sum/1 -> Gain/1
  Gain/1 -> A31/1
  normal(q)/1 -> Demux/1
  Demux/3 -> Product1/2
  Demux/2 -> Product2/1
  Demux/4 -> Product2/2
  Product2/1 -> Sum/2
  Product1/1 -> Sum/1
  Demux/1 -> Product1/1

== system ap_12BAdapted_with_contracts_AutoPilot/GlobalScope/DeHavilland Beaver Airframe/Aircraft Dynamics/6DoF (Quaternion)/Calculate DCM & Euler Angles/Quaternions to Direction Cosine Matrix/A32 ==
  normal(q) : Inport
  Demux : Demux
  Gain : Gain  Gain=2
  Product1 : Product  RndMeth=Zero
  Product2 : Product  RndMeth=Zero
  Sum : Sum  Inputs=|-+
  A32 : Outport  VectorParamsAs1DForOutWhenUnconnected=off
  wires:
  normal(q)/1 -> Demux/1
  Gain/1 -> A32/1
  Demux/3 -> Product2/1
  Demux/2 -> Product1/2
  Demux/1 -> Product1/1
  Sum/1 -> Gain/1
  Product1/1 -> Sum/1
  Product2/1 -> Sum/2
  Demux/4 -> Product2/2

== system ap_12BAdapted_with_contracts_AutoPilot/GlobalScope/DeHavilland Beaver Airframe/Aircraft Dynamics/6DoF (Quaternion)/Calculate DCM & Euler Angles/Quaternions to Direction Cosine Matrix/A33 ==
  normal(q) : Inport
  Demux : Demux
  Product{,1..3} (4 alike) : Product  RndMeth=Zero
  Sum : Sum  Inputs=+--+
  A33 : Outport  VectorParamsAs1DForOutWhenUnconnected=off
  wires:
  normal(q)/1 -> Demux/1
  Product/1 -> Sum/4
  Product1/1 -> Sum/3
  Product2/1 -> Sum/2
  Product3/1 -> Sum/1
  Demux/1 -> Product3/1, Product3/2
  Demux/2 -> Product2/1, Product2/2
  Demux/3 -> Product1/1, Product1/2
  Demux/4 -> Product/1, Product/2
  Sum/1 -> A33/1

== system ap_12BAdapted_with_contracts_AutoPilot/GlobalScope/DeHavilland Beaver Airframe/Aircraft Dynamics/6DoF (Quaternion)/Calculate DCM & Euler Angles/Quaternions to Direction Cosine Matrix/Create 3x3 Matrix ==
  M11 : Inport  PortDimensions=1
  M12 : Inport  Port=2  PortDimensions=1
  M13 : Inport  Port=3  PortDimensions=1
  M21 : Inport  Port=4  PortDimensions=1
  M22 : Inport  Port=5  PortDimensions=1
  M23 : Inport  Port=6  PortDimensions=1
  M31 : Inport  Port=7  PortDimensions=1
  M32 : Inport  Port=8  PortDimensions=1
  M33 : Inport  Port=9  PortDimensions=1
  Reshape (9) to [3x3] column-major : Reshape  OutputDimensionality=Customize  OutputDimensions=[3,3]
  Vector Concatenate : Concatenate  NumInputs=9
  Matrix : Outport  PortDimensions=[3 3]  VectorParamsAs1DForOutWhenUnconnected=off
  wires:
  M33/1 -> Vector Concatenate/9
  M23/1 -> Vector Concatenate/8
  M13/1 -> Vector Concatenate/7
  M32/1 -> Vector Concatenate/6
  Reshape (9) to [3x3] column-major/1 -> Matrix/1
  M22/1 -> Vector Concatenate/5
  M12/1 -> Vector Concatenate/4
  M31/1 -> Vector Concatenate/3
  M21/1 -> Vector Concatenate/2
  M11/1 -> Vector Concatenate/1
  Vector Concatenate/1 -> Reshape (9) to [3x3] column-major/1

== system ap_12BAdapted_with_contracts_AutoPilot/GlobalScope/DeHavilland Beaver Airframe/Aircraft Dynamics/6DoF (Quaternion)/Calculate DCM & Euler Angles/Quaternions to Direction Cosine Matrix/Quaternion Normalize ==
  q : Inport  Unit=1
  Demux : Demux
  Mux : Mux
  Product{,1..3} (4 alike) : Product  Inputs=*/
  Quaternion Modulus : Subsystem  mask(Quaternion Modulus){}
      mask help: shared_aeroblks:sharedaeroblkutil:blockQuaternionModulusDesc
      mask init:
      | if license('test','aerospace_blockset')
      |     aerosharedicon('shared');
      | elseif license('test','powertrain_blockset')
      |     sharedautoicon('shared');
      | end
      mask Help: eval('if license(''test'',''aerospace_blockset'')aerosharedhelp;elseif license(''test'',''powertrain_blockset'')sharedautohelp;end')
  normal(q) : Outport  Unit=1  VectorParamsAs1DForOutWhenUnconnected=off
  wires:
  Product3/1 -> Mux/4
  Product2/1 -> Mux/3
  Product1/1 -> Mux/2
  Product/1 -> Mux/1
  Quaternion Modulus/1(|q|) -> Product3/2, Product2/2, Product/2, Product1/2
  q/1 -> Demux/1, Quaternion Modulus/1(q)
  Mux/1 -> normal(q)/1
  Demux/1 -> Product/1
  Demux/2 -> Product1/1
  Demux/3 -> Product2/1
  Demux/4 -> Product3/1

== system ap_12BAdapted_with_contracts_AutoPilot/GlobalScope/DeHavilland Beaver Airframe/Aircraft Dynamics/6DoF (Quaternion)/Calculate DCM & Euler Angles/Quaternions to Rotation Angles (ZYX)/Quaternion Normalize ==
  q : Inport
  Demux : Demux
  Mux : Mux
  Product{,1..3} (4 alike) : Product  Inputs=*/
  Quaternion Modulus : Subsystem
  normal(q) : Outport  VectorParamsAs1DForOutWhenUnconnected=off
  wires:
  Product3/1 -> Mux/4
  Product1/1 -> Mux/2
  Demux/1 -> Product/1
  Quaternion Modulus/1(|q|) -> Product1/2, Product/2, Product2/2, Product3/2
  Mux/1 -> normal(q)/1
  q/1 -> Quaternion Modulus/1(q), Demux/1
  Product/1 -> Mux/1
  Demux/3 -> Product2/1
  Demux/4 -> Product3/1
  Product2/1 -> Mux/3
  Demux/2 -> Product1/1

== system ap_12BAdapted_with_contracts_AutoPilot/GlobalScope/DeHavilland Beaver Airframe/Aircraft Dynamics/6DoF (Quaternion)/Calculate omega_dot/3x3 CrossProduct/Subsystem ==
  A : Inport
  B : Inport  Port=2
  Demux : Demux  Outputs=3
  Demux1 : Demux  Outputs=3
  Mux : Mux  Inputs=3
  i x j : Product  SaturateOnIntegerOverflow=on  InputSameDT=on  OutDataTypeStr=Inherit: Same as first input
  j x k : Product  SaturateOnIntegerOverflow=on  InputSameDT=on  OutDataTypeStr=Inherit: Same as first input
  k x i : Product  SaturateOnIntegerOverflow=on  InputSameDT=on  OutDataTypeStr=Inherit: Same as first input
  Out1 : Outport  VectorParamsAs1DForOutWhenUnconnected=off
  wires:
  Demux1/3 -> j x k/2
  Demux/2 -> j x k/1
  Demux/3 -> k x i/1
  Demux1/1 -> k x i/2
  Demux1/2 -> i x j/2
  Demux/1 -> i x j/1
  i x j/1 -> Mux/3
  k x i/1 -> Mux/2
  j x k/1 -> Mux/1
  B/1 -> Demux1/1
  A/1 -> Demux/1
  Mux/1 -> Out1/1

== system ap_12BAdapted_with_contracts_AutoPilot/GlobalScope/DeHavilland Beaver Airframe/Aircraft Dynamics/6DoF (Quaternion)/Calculate omega_dot/3x3 CrossProduct/Subsystem1 ==
  A : Inport
  B : Inport  Port=2
  Demux : Demux  Outputs=3
  Demux1 : Demux  Outputs=3
  Mux : Mux  Inputs=3
  i x k : Product  SaturateOnIntegerOverflow=on  InputSameDT=on  OutDataTypeStr=Inherit: Same as first input
  j x i : Product  SaturateOnIntegerOverflow=on  InputSameDT=on  OutDataTypeStr=Inherit: Same as first input
  k x j : Product  SaturateOnIntegerOverflow=on  InputSameDT=on  OutDataTypeStr=Inherit: Same as first input
  Out1 : Outport  VectorParamsAs1DForOutWhenUnconnected=off
  wires:
  j x i/1 -> Mux/3
  i x k/1 -> Mux/2
  k x j/1 -> Mux/1
  Mux/1 -> Out1/1
  Demux1/1 -> j x i/2
  Demux/2 -> j x i/1
  Demux1/3 -> i x k/2
  Demux/1 -> i x k/1
  Demux1/2 -> k x j/2
  Demux/3 -> k x j/1
  B/1 -> Demux1/1
  A/1 -> Demux/1

== system ap_12BAdapted_with_contracts_AutoPilot/GlobalScope/DeHavilland Beaver Airframe/Aircraft Dynamics/Total Forces and Moments/Actuators/sof/ResetIntegratorInternal ==
  note: ic
  note: Level Reset Integration With Saturation
      | y(n) = y(n-1) + K*Ts*u(n-1)
  U : Inport
  R : Inport  Port=2
  ic : Inport  Port=3
  Constant : Constant  Value=1.0
  Constant1 : Constant  Value=Ts
  Product : Product  RndMeth=Zero
  Product1 : Product  RndMeth=Zero
  Sum3 : Sum
  Switch : Switch  Criteria=u2 ~= 0
  Switch1 : Switch  Criteria=u2 ~= 0
  X : UnitDelay  SampleTime=Ts  HasFrameUpgradeWarning=on
  Y : Outport  VectorParamsAs1DForOutWhenUnconnected=off
  wires:
  Product1/1 -> Sum3/1
  U/1 -> Product1/2
  Sum3/1 -> Switch1/3
  Product/1 -> Product1/1
  ic/1 -> Switch1/1, Switch/1
  Constant1/1 -> Product/2  "deltaT"
  Switch1/1 -> X/1
  Constant/1 -> Product/1  "gain"
  Switch/1 -> Y/1, Sum3/2
  R/1 -> Switch1/2, Switch/2
  X/1 -> Switch/3

== system ap_12BAdapted_with_contracts_AutoPilot/GlobalScope/DeHavilland Beaver Airframe/Aircraft Dynamics/Total Forces and Moments/Actuators/sof/ResetIntegratorInternal1 ==
  note: Level Reset Integration With Saturation
      | y(n) = y(n-1) + K*Ts*u(n-1)
  note: ic
  U : Inport
  R : Inport  Port=2
  ic : Inport  Port=3
  Constant : Constant  Value=1.0
  Constant1 : Constant  Value=Ts
  Product : Product  RndMeth=Zero
  Product1 : Product  RndMeth=Zero
  Saturation : Saturate  UpperLimit=fin_max  LowerLimit=fin_min
  Sum3 : Sum
  Switch : Switch  Criteria=u2 ~= 0
  Switch1 : Switch  Criteria=u2 ~= 0
  X : UnitDelay  SampleTime=Ts  HasFrameUpgradeWarning=on
  Y : Outport  VectorParamsAs1DForOutWhenUnconnected=off
  wires:
  X/1 -> Switch/3
  R/1 -> Switch/2, Switch1/2
  Saturation/1 -> Sum3/2, Y/1
  Constant/1 -> Product/1  "gain"
  Switch1/1 -> X/1
  Constant1/1 -> Product/2  "deltaT"
  ic/1 -> Switch/1, Switch1/1
  Switch/1 -> Saturation/1
  Product/1 -> Product1/1
  Sum3/1 -> Switch1/3
  U/1 -> Product1/2
  Product1/1 -> Sum3/1

== system ap_12BAdapted_with_contracts_AutoPilot/GlobalScope/DeHavilland Beaver Airframe/Aircraft Dynamics/Total Forces and Moments/Actuators/sof/ic1 ==
  Constant : Constant  Value=0
  Constant1 : Constant  Value=fin_act_1
  Unit Delay : UnitDelay  InitialCondition=1  SampleTime=-1  HasFrameUpgradeWarning=on
  R : Outport  VectorParamsAs1DForOutWhenUnconnected=off
  IC : Outport  Port=2  VectorParamsAs1DForOutWhenUnconnected=off
  wires:
  Constant1/1 -> IC/1
  Unit Delay/1 -> R/1
  Constant/1 -> Unit Delay/1

== system ap_12BAdapted_with_contracts_AutoPilot/GlobalScope/DeHavilland Beaver Airframe/Aircraft Dynamics/Total Forces and Moments/Actuators/sof/ic3 ==
  Constant : Constant  Value=0
  Constant1 : Constant  Value=0.0
  Unit Delay : UnitDelay  InitialCondition=1  SampleTime=-1  HasFrameUpgradeWarning=on
  R : Outport  VectorParamsAs1DForOutWhenUnconnected=off
  IC : Outport  Port=2  VectorParamsAs1DForOutWhenUnconnected=off
  wires:
  Constant/1 -> Unit Delay/1
  Unit Delay/1 -> R/1
  Constant1/1 -> IC/1

== system ap_12BAdapted_with_contracts_AutoPilot/GlobalScope/DeHavilland Beaver Airframe/Aircraft Dynamics/Total Forces and Moments/Actuators/sof1/ResetIntegratorInternal ==
  note: Level Reset Integration With Saturation
      | y(n) = y(n-1) + K*Ts*u(n-1)
  note: ic
  U : Inport
  R : Inport  Port=2
  ic : Inport  Port=3
  Constant : Constant  Value=1.0
  Constant1 : Constant  Value=Ts
  Product : Product  RndMeth=Zero
  Product1 : Product  RndMeth=Zero
  Sum3 : Sum
  Switch : Switch  Criteria=u2 ~= 0
  Switch1 : Switch  Criteria=u2 ~= 0
  X : UnitDelay  SampleTime=Ts  HasFrameUpgradeWarning=on
  Y : Outport  VectorParamsAs1DForOutWhenUnconnected=off
  wires:
  X/1 -> Switch/3
  R/1 -> Switch/2, Switch1/2
  Switch/1 -> Sum3/2, Y/1
  Constant/1 -> Product/1  "gain"
  Switch1/1 -> X/1
  Constant1/1 -> Product/2  "deltaT"
  ic/1 -> Switch/1, Switch1/1
  Product/1 -> Product1/1
  Sum3/1 -> Switch1/3
  U/1 -> Product1/2
  Product1/1 -> Sum3/1

== system ap_12BAdapted_with_contracts_AutoPilot/GlobalScope/DeHavilland Beaver Airframe/Aircraft Dynamics/Total Forces and Moments/Actuators/sof1/ResetIntegratorInternal1 ==
  note: ic
  note: Level Reset Integration With Saturation
      | y(n) = y(n-1) + K*Ts*u(n-1)
  U : Inport
  R : Inport  Port=2
  ic : Inport  Port=3
  Constant : Constant  Value=1.0
  Constant1 : Constant  Value=Ts
  Product : Product  RndMeth=Zero
  Product1 : Product  RndMeth=Zero
  Saturation : Saturate  UpperLimit=fin_max  LowerLimit=fin_min
  Sum3 : Sum
  Switch : Switch  Criteria=u2 ~= 0
  Switch1 : Switch  Criteria=u2 ~= 0
  X : UnitDelay  SampleTime=Ts  HasFrameUpgradeWarning=on
  Y : Outport  VectorParamsAs1DForOutWhenUnconnected=off
  wires:
  Product1/1 -> Sum3/1
  U/1 -> Product1/2
  Sum3/1 -> Switch1/3
  Product/1 -> Product1/1
  Switch/1 -> Saturation/1
  ic/1 -> Switch1/1, Switch/1
  Constant1/1 -> Product/2  "deltaT"
  Switch1/1 -> X/1
  Constant/1 -> Product/1  "gain"
  Saturation/1 -> Y/1, Sum3/2
  R/1 -> Switch1/2, Switch/2
  X/1 -> Switch/3

== system ap_12BAdapted_with_contracts_AutoPilot/GlobalScope/DeHavilland Beaver Airframe/Aircraft Dynamics/Total Forces and Moments/Actuators/sof1/ic1 ==
  Constant : Constant  Value=0
  Constant1 : Constant  Value=fin_act_2
  Unit Delay : UnitDelay  InitialCondition=1  SampleTime=-1  HasFrameUpgradeWarning=on
  R : Outport  VectorParamsAs1DForOutWhenUnconnected=off
  IC : Outport  Port=2  VectorParamsAs1DForOutWhenUnconnected=off
  wires:
  Constant/1 -> Unit Delay/1
  Unit Delay/1 -> R/1
  Constant1/1 -> IC/1

== system ap_12BAdapted_with_contracts_AutoPilot/GlobalScope/DeHavilland Beaver Airframe/Aircraft Dynamics/Total Forces and Moments/Actuators/sof1/ic3 ==
  Constant : Constant  Value=0
  Constant1 : Constant  Value=0.0
  Unit Delay : UnitDelay  InitialCondition=1  SampleTime=-1  HasFrameUpgradeWarning=on
  R : Outport  VectorParamsAs1DForOutWhenUnconnected=off
  IC : Outport  Port=2  VectorParamsAs1DForOutWhenUnconnected=off
  wires:
  Constant1/1 -> IC/1
  Unit Delay/1 -> R/1
  Constant/1 -> Unit Delay/1

== system ap_12BAdapted_with_contracts_AutoPilot/GlobalScope/DeHavilland Beaver Airframe/Aircraft Dynamics/Total Forces and Moments/Actuators/sof2/ResetIntegratorInternal ==
  note: ic
  note: Level Reset Integration With Saturation
      | y(n) = y(n-1) + K*Ts*u(n-1)
  U : Inport
  R : Inport  Port=2
  ic : Inport  Port=3
  Constant : Constant  Value=1.0
  Constant1 : Constant  Value=Ts
  Product : Product  RndMeth=Zero
  Product1 : Product  RndMeth=Zero
  Sum3 : Sum
  Switch : Switch  Criteria=u2 ~= 0
  Switch1 : Switch  Criteria=u2 ~= 0
  X : UnitDelay  SampleTime=Ts  HasFrameUpgradeWarning=on
  Y : Outport  VectorParamsAs1DForOutWhenUnconnected=off
  wires:
  Product1/1 -> Sum3/1
  U/1 -> Product1/2
  Sum3/1 -> Switch1/3
  Product/1 -> Product1/1
  ic/1 -> Switch1/1, Switch/1
  Constant1/1 -> Product/2  "deltaT"
  Switch1/1 -> X/1
  Constant/1 -> Product/1  "gain"
  Switch/1 -> Y/1, Sum3/2
  R/1 -> Switch1/2, Switch/2
  X/1 -> Switch/3

== system ap_12BAdapted_with_contracts_AutoPilot/GlobalScope/DeHavilland Beaver Airframe/Aircraft Dynamics/Total Forces and Moments/Actuators/sof2/ResetIntegratorInternal1 ==
  note: Level Reset Integration With Saturation
      | y(n) = y(n-1) + K*Ts*u(n-1)
  note: ic
  U : Inport
  R : Inport  Port=2
  ic : Inport  Port=3
  Constant : Constant  Value=1.0
  Constant1 : Constant  Value=Ts
  Product : Product  RndMeth=Zero
  Product1 : Product  RndMeth=Zero
  Saturation : Saturate  UpperLimit=fin_max  LowerLimit=fin_min
  Sum3 : Sum
  Switch : Switch  Criteria=u2 ~= 0
  Switch1 : Switch  Criteria=u2 ~= 0
  X : UnitDelay  SampleTime=Ts  HasFrameUpgradeWarning=on
  Y : Outport  VectorParamsAs1DForOutWhenUnconnected=off
  wires:
  X/1 -> Switch/3
  R/1 -> Switch/2, Switch1/2
  Saturation/1 -> Sum3/2, Y/1
  Constant/1 -> Product/1  "gain"
  Switch1/1 -> X/1
  Constant1/1 -> Product/2  "deltaT"
  ic/1 -> Switch/1, Switch1/1
  Switch/1 -> Saturation/1
  Product/1 -> Product1/1
  Sum3/1 -> Switch1/3
  U/1 -> Product1/2
  Product1/1 -> Sum3/1

== system ap_12BAdapted_with_contracts_AutoPilot/GlobalScope/DeHavilland Beaver Airframe/Aircraft Dynamics/Total Forces and Moments/Actuators/sof2/ic1 ==
  Constant : Constant  Value=0
  Constant1 : Constant  Value=fin_act_3
  Unit Delay : UnitDelay  InitialCondition=1  SampleTime=-1  HasFrameUpgradeWarning=on
  R : Outport  VectorParamsAs1DForOutWhenUnconnected=off
  IC : Outport  Port=2  VectorParamsAs1DForOutWhenUnconnected=off
  wires:
  Constant1/1 -> IC/1
  Unit Delay/1 -> R/1
  Constant/1 -> Unit Delay/1

== system ap_12BAdapted_with_contracts_AutoPilot/GlobalScope/DeHavilland Beaver Airframe/Aircraft Dynamics/Total Forces and Moments/Actuators/sof2/ic3 ==
  Constant : Constant  Value=0
  Constant1 : Constant  Value=0.0
  Unit Delay : UnitDelay  InitialCondition=1  SampleTime=-1  HasFrameUpgradeWarning=on
  R : Outport  VectorParamsAs1DForOutWhenUnconnected=off
  IC : Outport  Port=2  VectorParamsAs1DForOutWhenUnconnected=off
  wires:
  Constant/1 -> Unit Delay/1
  Unit Delay/1 -> R/1
  Constant1/1 -> IC/1

== system ap_12BAdapted_with_contracts_AutoPilot/GlobalScope/DeHavilland Beaver Airframe/Aircraft Dynamics/Total Forces and Moments/Aerodynamics/Actuator Increments/Aileron ==
  alpha : Inport
  Actuators : Inport  Port=2
  Gain1 : Gain  Gain=0  SaturateOnIntegerOverflow=on  OutDataTypeStr=Inherit: Same as input  ParamDataTypeStr=Inherit: Same as input
  Gain2 : Gain  Gain=Cy_da  SaturateOnIntegerOverflow=on  OutDataTypeStr=Inherit: Same as input  ParamDataTypeStr=Inherit: Same as input
  Gain3 : Gain  Gain=0  SaturateOnIntegerOverflow=on  OutDataTypeStr=Inherit: Same as input  ParamDataTypeStr=Inherit: Same as input
  Gain4 : Gain  Gain=Cn_da  SaturateOnIntegerOverflow=on  OutDataTypeStr=Inherit: Same as input  ParamDataTypeStr=Inherit: Same as input
  Gain5 : Gain  Gain=0  SaturateOnIntegerOverflow=on  OutDataTypeStr=Inherit: Same as input  ParamDataTypeStr=Inherit: Same as input
  Gain6 : Gain  Gain=Cl_da  SaturateOnIntegerOverflow=on  OutDataTypeStr=Inherit: Same as input  ParamDataTypeStr=Inherit: Same as input
  Gain7 : Gain  Gain=Cl_da_alpha  SaturateOnIntegerOverflow=on  OutDataTypeStr=Inherit: Same as input  ParamDataTypeStr=Inherit: Same as input
  Mux1 : Mux  Inputs=6
  Product4 : Product  SaturateOnIntegerOverflow=on  InputSameDT=on  OutDataTypeStr=Inherit: Same as first input
  Selector1 : Selector  InputPortWidth=4  IndexOptions=Index vector (dialog)  Indices=2  OutputSizes=1
  Sum1 : Sum  Inputs=++|  SaturateOnIntegerOverflow=on
  delCoeff : Outport  VectorParamsAs1DForOutWhenUnconnected=off
  wires:
  Gain6/1 -> Sum1/1
  Sum1/1 -> Mux1/4
  Gain7/1 -> Sum1/2
  Product4/1 -> Gain7/1
  Gain1/1 -> Mux1/1  "Cx"
  alpha/1 -> Product4/2
  Actuators/1 -> Selector1/1
  Mux1/1 -> delCoeff/1
  Gain2/1 -> Mux1/2  "Cy"
  Gain3/1 -> Mux1/3  "Cz"
  Gain5/1 -> Mux1/5  "Cm"
  Gain4/1 -> Mux1/6
  Selector1/1 -> Gain1/1, Gain2/1, Gain3/1, Gain6/1, Product4/1, Gain5/1, Gain4/1
